simulink model "Copy_of_fast_powertrain"  (R2020b)
settings: Solver=FixedStepAuto  StartTime=0  StopTime=t(end)  RelTol=1e-3
PreLoadFcn:
  | C_sc = 1;
StartFcn:
  | C_sc = 1;
values from neighbouring files (symbols this model uses):
  fc_power_array = [900 900 900 900 900 900 900 900 900 900 900 900 ... (24566 elements, 71x346)]    [fc_power_climb_dp.mat]    (also in fc_power_cruise_dp.mat = [0 0 0 0 0 0 0 0 0 0 0 0 ... (32589 elements, 71x459)]; fc_power_descend_dp.mat = [285.411057245 285.411057245 285.411057245 285.411057245 285; fc_power_takeoff_dp.mat = [0 0 0 0 0 0 0 0 0 0 0 0 ... (23714 elements, 71x334)])
  Ts = old_data.Ts    [model_fc.m]
undefined symbols (not defined in the file or in its folder): DiscIntNeverNeededParam, Ion, Lithium, w
libraries: neural x50, powerlib x30, fuzblock x7, electricdrivelib x2, lib_converters x2, simulink x1
(part 1 of 5)
PostSaveFcn:
  | C_sc = 1;
settings Model: SimulationMode=accelerator  Creator=maloc  LastModifiedBy=maloc
settings DataIOCC: SaveOutput=off  SignalLogging=off  DSMLogging=off
settings OptimizationCC: StrengthReduction=on  PassReuseOutputArgsAs=Individual arguments  LocalBlockOutputs=off  ZeroExternalMemoryAtStartup=off  ZeroInternalMemoryAtStartup=off  OptimizeBlockOrder=speed  OptimizationPriority=Speed  MultiThreadedLoops=on  EfficientTunableParamExpr=on
settings DebuggingCC: RTPrefix=none  StringTruncationChecking=none  AlgebraicLoopMsg=none  ArtificialAlgebraicLoopMsg=none  MaxConsecutiveZCsMsg=none  InheritedTsInSrcMsg=none  MultiTaskDSMMsg=none  MultiTaskCondExecSysMsg=none  MultiTaskRateTransMsg=warning  TasksWithSamePriorityMsg=none  SigSpecEnsureSampleTimeMsg=none  IntegerOverflowMsg=none  Int32ToFloatConvMsg=none  ParameterDowncastMsg=none  ParameterOverflowMsg=none  ParameterPrecisionLossMsg=none  ParameterTunabilityLossMsg=none  FcnCallInpInsideContextMsg=warning  UnconnectedInputMsg=none  UnconnectedOutputMsg=none  UnconnectedLineMsg=none  FrameProcessingCompatibilityMsg=none  BusObjectLabelMismatch=none  RootOutportRequireBusObject=none  UnknownTsInhSupMsg=none  ModelReferenceDataLoggingMessage=none  ModelReferenceExtraNoncontSigs=none  OperatingPointInterfaceChecksumMismatchMsg=none  NonCurrentReleaseOperatingPointMsg=warning  SFUnexpectedBacktrackingDiag=warning  SFNoUnconditionalDefaultTransitionDiag=warning  IntegerSaturationMsg=none
settings SFSimCC: MATLABDynamicMemAlloc=off  SimTargetLang=C++
settings RTWCC: Description=Embedded Coder  SystemTargetFile=ert.tlc  GenCodeOnly=on  TemplateMakefile=ert_default_tmf  GenerateReport=on  BuildConfiguration=Debug  LaunchReport=on
settings CodeAppCC: ForceParamTrailComments=on  IgnoreCustomStorageClasses=off  OperatorAnnotations=on  SimulinkDataObjDesc=on  SFDataObjDesc=on  InsertBlockDesc=on  EnableCustomComments=on
settings ERTTargetCC: TargetLangStandard=C99 (ISO)  GenerateSampleERTMain=on  ERTCustomFileTemplate=example_file_process.tlc

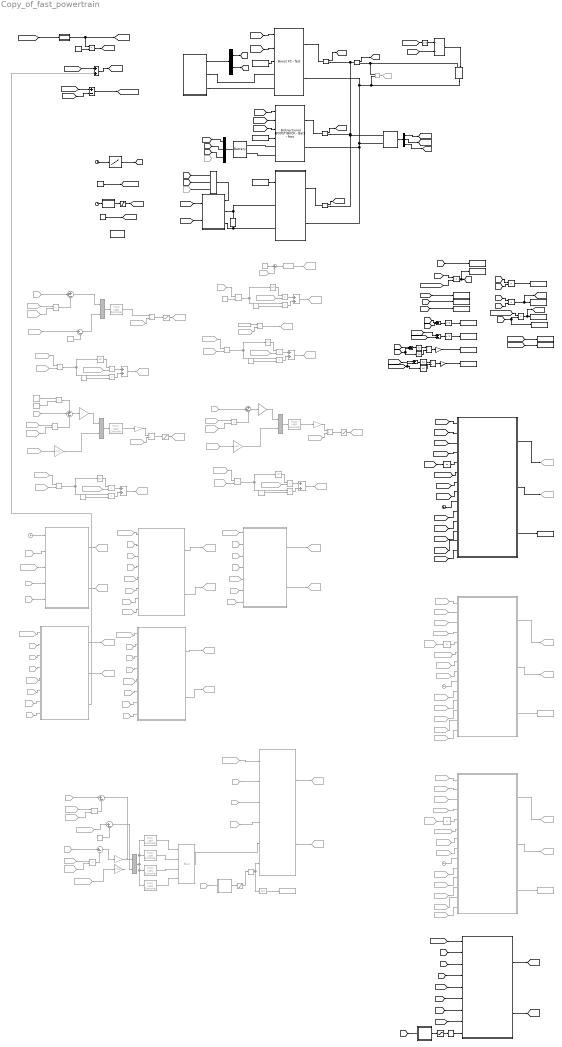
== system Copy_of_fast_powertrain ==
  note: GA
  note: DP-ANFIS
  note: Pload
  note: Data
  note: Powertrain
  note: Load
  note: Inputs
  note: BATT Control
  note: PV - FC Control
  note: PV Panel weather data
  note: ANFIS+NN
  1-D Lookup Table1 : Lookup_n-D  NumberOfTableDimensions=1  BreakpointsForDimension1=t  Table=w  InternalRulePriority=Speed  RndMeth=Simplest  InputSameDT=on
  Abs{,1..3} (4 alike) : Abs
  Battery : electricdrivelib/Extra Sources/Battery  BatType=Lithium-Ion  ShowTempParam=off  ThermalPreset=no  ShowAgeParam=off  NomV=48  NomQ=15  SOC=80  Batt_Tr=20  PresetModel=on  MaxQ=15  MinV=36  FullV=55.8714  Dis_rate=6.5217  R=0.032  Normal_OP=13.5652  expZone="[51.8585     0.736957]"  current=[2 5 10 40]  Units=Time  Tci=20  NomT=20  T2=-30  MaxQ2=4.8  FullV2=7.1  Normal_OP2=5.655  expZone2="[6.58           1]"  Rca=0.6  ti=2000  Dp=0  Neq0=0  Tsim=Ts  Ta1=25  Qeol=5.4*0.9  Reol=0.013333*1.2  Char_age=[2.3478, 3]  Dis_age=[2.3478, 10]  N1=1500  N2=10500  N3=1000  N4=1400  Ta2=45  N5=950
      link override Model/Constant15: Value=Batt_Tr
  Bidirectional BOOST/BUCK - Batt - fast : lib_converters/Bidirectional BOOST//BUCK - Batt - fast  n_buck=0.9  Tr_buck=1  damp_buck=0.707  n_boost=0.9  Tr_boost=1  damp_boost=0.707  max_curr=[30 -4]  Co=1e-4  CL=C_sc  Li=1e-3  Ts=Ts
  Boost - PV - fast : Subsystem  AncestorBlock=lib_converters/Boost - PV - fast  mask(Average value DC/DC boost converter for PV panel){n=0.9, Co=1e-4, CL=C_sc, Li=2e-3, damp=0.707, Tr=0.1, Ts=Ts}
      mask prompts: n "Efficiency [0,1]"; Co "Inside output capacitance (F)"; CL "Load Capacitance (F)"; Li "Input Inductor (H)"; damp "Damping ratio"; Tr "Response time (s) (Voltage Regulator)"; Ts "Sample time (s)"
      mask help:
      | This block implements an average-value DC/DC boost converter.
      | - VH* input is the control variable of the output voltage of the converter.
      | - IL*(max) input is the control variable of the input max current of the converter.
      | - I/O input control the converter to enable it to work or not (interruptor control command).
      | - Control input is the variable that manage the control strategy of the converter (MPPT, Cascade control, ...).
      mask init:
      | L=Li; 
      | C=Co+CL;
      | 
      | %Current regulator
      | zetai=damp;
      | thau_si=Tr/10;
      | zetawni=(-log(0.05*sqrt(1-zetai^2)))/thau_si;
      | Kpi=2*L*zetawni;
      | wni=zetawni/zetai;
      | Kii=L*wni^2;
      | 
      | %Voltage regulator
      | zetav=damp;
      | thau_sv=Tr; %response time
      | zetawnv=(-log(0.05*sqrt(1-zetav^2)))/thau_sv;
      | Kpv=2*C*zetawnv;
      | wnv=zetawnv/zetav;
      | Kiv=C*wnv^2;
      mask Help:
      | 1 - MPPT
      | 2 - Cascade control
  Boost FC - fast : lib_converters/Boost FC - fast  conv_type=Average model  n=0.9  Co=1e-4  CL=C_sc  Li=2e-3  damp=0.707  Tr=1  Ts=Ts
  Bus Selector : BusSelector  OutputSignals=SOC (%),Current (A),Voltage (V)
  Bus Selector1 : BusSelector  OutputSignals=Current I,SOC %,Voltage V
  Bus Selector2 : BusSelector  OutputSignals=Vout,Ifc
  Bus Selector3 : BusSelector  OutputSignals=V_PV,I_PV,Temperature (deg C)
  C2 : powerlib/Elements/Series RLC Branch  LConnTagsString=__new0  RConnTagsString=__new0  BranchType=C  Resistance=0.01  Inductance=1e-3  SetiL0=off  InitialCurrent=0  Capacitance=1e-3  Setx0=off  InitialVoltage=0  Measurements=None
  Clock : Clock  Commented=on
  Clock1 : Clock
  Clock2 : Clock  Commented=on
  Clock3 : Clock  Commented=on
  Clock4 : Clock
  Clock6 : Clock
  Constant : Constant  Commented=on  Value=20
  Constant1 : Constant
  Constant10 : Constant  Commented=on  Value=80
  Constant{4,11,13,17,19} (5 alike) : Constant  Commented=on  Value=100
  Constant14 : Constant  Commented=on  Value=20
  Constant15 : Constant  Commented=on  Value=180
  Constant16 : Constant  Commented=on  Value=0.9
  Constant2 : Constant
  Constant3 : Constant
  Constant5 : Constant  Commented=on  Value=580
  Constant6 : Constant  Value=72
  Constant7 : Constant  Commented=on  Value=80
  Constant8 : Constant  Value=0
  Constant9 : Constant  Value=25
  Current Measurement{,2..4} (4 alike) : powerlib/Measurements/Current Measurement  PhasorSimulation=off  OutputType=Complex  PSBequivalent=0
  DP : MATLAB Function  Commented=on  TreatAsAtomicUnit=on  mask{fc_power_array=fc_power_array}
  Discrete PI Controller1 : Subsystem  Commented=on  DialogController=POWERSYS.PowerSysDialog  mask(Discrete PI Controller){Kp=10, Ki=10, Par_Limits=[33 0], Init=0, Ts=Ts}
      mask prompts: Kp "Proportional gain (Kp):"; Ki "Integral gain (Ki):"; Par_Limits "Output limits: [ Upper   Lower ]"; Init "Output initial value:"; Ts "Sample time:"
      mask help: This block implements a discrete PI controller.
      mask init:
      | UpperLimit=Par_Limits(1);
      | LowerLimit=Par_Limits(2);
      | power_initmask();
      mask Help: This block is part of a subset of blocks in the Extras library that does not have documentation associated with it, other than the block mask description.
      mask Display: disp('PI');
  Discrete PI Controller2 : Subsystem  DialogController=POWERSYS.PowerSysDialog  mask(Discrete PI Controller){Kp=10, Ki=100, Par_Limits=[30 -4], Init=0, Ts=Ts}
      mask prompts: Kp "Proportional gain (Kp):"; Ki "Integral gain (Ki):"; Par_Limits "Output limits: [ Upper   Lower ]"; Init "Output initial value:"; Ts "Sample time:"
      mask help: This block implements a discrete PI controller.
      mask init:
      | UpperLimit=Par_Limits(1);
      | LowerLimit=Par_Limits(2);
      | power_initmask();
      mask Help: This block is part of a subset of blocks in the Extras library that does not have documentation associated with it, other than the block mask description.
      mask Display: disp('PI');
  Divide : Product  Inputs=*/
  Divide{1,4..6} (4 alike) : Product  Commented=on  Inputs=*/
  Divide2 : Product  Inputs=*/
  Divide3 : Product  Inputs=*/
  ECMS : MATLAB Function  Commented=on  TreatAsAtomicUnit=on
  EEDMS : MATLAB Function  Commented=on  TreatAsAtomicUnit=on
  EEMS : MATLAB Function  Commented=on  TreatAsAtomicUnit=on
  From100 : From  Commented=on  GotoTag=Vbus_real
  From{4,25,41,47,50,58,68,78,86,94,101,110,141} (13 alike) : From  Commented=on  GotoTag=V_dc_bus_wanted
  From{3,27,48,52,59,69,79,87,95,102,120,149} (12 alike) : From  Commented=on  GotoTag=V_fc
  From{26,38,49,53,60,70,76,84,92,103,118,123,147,150} (14 alike) : From  Commented=on  GotoTag=I_fc
  From{43,57,65,74,83,91,104,111,137,142} (10 alike) : From  Commented=on  GotoTag=V_dc_bus
  From105 : From  Commented=on  GotoTag=Vbus_real
  From106 : From  Commented=on  GotoTag=BATT_SOC
  From{39,54,61,71,81,89,96,98,107,113,139,152} (12 alike) : From  Commented=on  GotoTag=Pload
  From108 : From  Commented=on  GotoTag=Ipv_out
  From{42,56,64,73,82,90,109,136,140} (9 alike) : From  Commented=on  GotoTag=I_pv_out
  From{13,35,40,51,55,63,72,80,88,112,116,145} (12 alike) : From  Commented=on  GotoTag=SOC_batt
  From114 : From  Commented=on  GotoTag=I_fc_out
  From{34,77,85,93,115,144} (6 alike) : From  Commented=on  GotoTag=I_fc_conv
  From117 : From  Commented=on  GotoTag=Pfc_in
  From{66,75,119,148} (4 alike) : From  Commented=on  GotoTag=I_batt
  From138 : From  Commented=on  GotoTag=Pout
  From143 : From  Commented=on  GotoTag=I_fc_out
  From146 : From  Commented=on  GotoTag=Pfc_in
  From151 : From  Commented=on  GotoTag=Pout
  From67 : From  Commented=on  GotoTag=Pbatt_in
  From97 : From  Commented=on  GotoTag=BATT_SOC
  From99 : From  Commented=on  GotoTag=Ipv_out
  Fuzzy Logic Controller : fuzblock/Fuzzy Logic  Controller  Commented=on  FIS='DP_ANFIS_mid.fis'  OutputSampleNumber=10  DataType=double  FuzzifiedInputs=off  RuleFiringStrengths=off  RuleOutputs=off  AggregatedOutputs=off  SimulateUsing=Code generation  OutOfRangeInputValueMessage=warning  NoRuleFiredMessage=warning  EmptyOutputFuzzySetMessage=warning
  Fuzzy Logic Controller1 : fuzblock/Fuzzy Logic  Controller  Commented=on  FIS='fuzzy_for_final_1.fis'  OutputSampleNumber=10  DataType=double  FuzzifiedInputs=off  RuleFiringStrengths=off  RuleOutputs=off  AggregatedOutputs=off  SimulateUsing=Code generation  OutOfRangeInputValueMessage=warning  NoRuleFiredMessage=warning  EmptyOutputFuzzySetMessage=warning
  Fuzzy Logic Controller2 : fuzblock/Fuzzy Logic  Controller  Commented=on  FIS='fis_thesis_solo.fis'  OutputSampleNumber=10  DataType=double  FuzzifiedInputs=off  RuleFiringStrengths=off  RuleOutputs=off  AggregatedOutputs=off  SimulateUsing=Code generation  OutOfRangeInputValueMessage=warning  NoRuleFiredMessage=warning  EmptyOutputFuzzySetMessage=warning
  Goto{13,25,28,30,32,34,39..41,44,47,49,51,55} (14 alike) : Goto  Commented=on  GotoTag=V_fc_conv
  Goto{7,24,27,29,31,33,37,42..43,45..46,48,50,54} (14 alike) : Goto  Commented=on  GotoTag=I_fc_conv
  Goto36 : Goto  Commented=on  GotoTag=T_pv
  Goto38 : Goto  Commented=on  GotoTag=Age
  Goto53 : Goto  Commented=on  GotoTag=V_dc_bus
  GreaterThan{,2..5} (5 alike) : RelationalOperator  Commented=on  Operator=<  OutDataTypeStr=boolean  RndMeth=Simplest
  GreaterThan1 : RelationalOperator  Operator=<  OutDataTypeStr=boolean  RndMeth=Simplest
  LMC : MATLAB Function  TreatAsAtomicUnit=on
  LMC-deep : MATLAB Function  Commented=on  TreatAsAtomicUnit=on
  LMC-deep1 : MATLAB Function  Commented=on  TreatAsAtomicUnit=on
  Multiply : Gain  Gain=100
  Multiply1 : Gain  Gain=100
  Multiply2 : Gain  Commented=on  Gain=1/1550
  Multiply3 : Gain  Commented=on  Gain=1/100
  Multiply4 : Gain  Commented=on  Gain=1100
  Multiply5 : Gain  Commented=on  Gain=1/1550
  Multiply6 : Gain  Commented=on  Gain=1/100
  Multiply7 : Gain  Commented=on  Gain=1100
  Multiply8 : Gain  Commented=on  Gain=1/1500
  Multiply9 : Gain  Commented=on  Gain=1/100
  Mux{,1..3} (4 alike) : Mux  Commented=on  Inputs=2
  Mux4 : Mux  Commented=on
      settings: DisplayOption=signals
  NN-SMC : MATLAB Function  TreatAsAtomicUnit=on
  NOT{,1..4} (5 alike) : Logic  Commented=on  Operator=NOT  IconShape=distinctive  AllPortsSameDT=off  OutDataTypeStr=boolean
  PEMFC matfunc V1 : Subsystem  mask{P_H2=0.5, P_O2=1, T=313.15, W=14, tm=1.27e-4, Nfc=50, Rohm=0.061871, Ts=Ts, fc_tau=1}
      mask prompts: P_H2 "Hydrogen pressure (atm)"; P_O2 "Oxygen pressure (atm)"; T "Temperature (K)"; W "Water Content"; tm "Thickness of the membrane (m)"; Nfc "Number of cells"; Rohm "Fuel cell resistance"; Ts "Sample time (s)"; fc_tau "Dynamic response of the FC (s)"
      mask init:
      | tau = fc_tau / 5;
  PV - FC - control1 : MATLAB Function  Commented=on  TreatAsAtomicUnit=on
  PV MODULE2 : Subsystem  mask{Npar=1, Nser=1, Ncell=72, Pm=0, Voc=44.5, Isc=5.54, Vmpp=37.2, Impp=4.97, beta_Voc_pc=-0.34, alpha_Isc_pc=-0.017, beta_Voc=0, alpha_Isc=0, IL=5.55564, I0=2.39143e-10, df=0.96618, Rsh=113.762, Rs=0.32122, Ts=Ts}
      mask prompts: Npar "Parallel connected modules"; Nser "Series connected modules"; Ncell "Number of cells per module"; Pm "Maxium Power (W)"; Voc "Open circuit voltage Voc (V)"; Isc "Short-circuit current Isc (A)"; Vmpp "Voltage at MPP (V)"; Impp "Current at MPP (A)"; beta_Voc_pc "Temperature coefficient of Voc (%/deg.C"; alpha_Isc_pc "Temperature coefficient of Isc (%/deg.C)"; beta_Voc "Temperature coefficient of Voc (V/deg.C)"; alpha_Isc "Temperature coefficient of Isc (A/deg.C)"; IL "Light-generated current IL (A)"; I0 "Diode saturation current I0 (A)"; df "Diode ideality factor"; Rsh "Shunt resistance Rsh (ohms)"; Rs "Series resistance Rs (ohms)"; Ts "Sample time (s)"
      mask init:
      | if alpha_Isc ~= 0
      |     alpha = alpha_Isc;
      | else 
      |     alpha = alpha_Isc_pc * Isc/100;
      | end
      mask DialogControl Container5 Prompt: Module data
      mask DialogControl Container3 Prompt: Data from data sheet
      mask DialogControl Container6 Prompt: Data from NREL
  Product{,1,4,7} (4 alike) : Product
  Product{2..3,5..6,8..18,21} (16 alike) : Product  Commented=on
  Round : Rounding  Commented=on  Operator=round
  Round1 : Rounding  Operator=round
  SMC : MATLAB Function  Commented=on  TreatAsAtomicUnit=on
  Saturation : Saturate  UpperLimit=1000  LowerLimit=0
  Saturation1 : Saturate  Commented=on  UpperLimit=1100  LowerLimit=0
  Saturation2 : Saturate  Commented=on  UpperLimit=1100  LowerLimit=0
  Saturation3 : Saturate  Commented=on  UpperLimit=1100  LowerLimit=0
  Saturation4 : Saturate  Commented=on  UpperLimit=4  LowerLimit=1
  Saturation5 : Saturate  UpperLimit=4  LowerLimit=1
  Square : Math  Operator=square  SaturateOnIntegerOverflow=on
  Square1 : Math  Operator=square  SaturateOnIntegerOverflow=on
  Square2 : Math  Operator=square  SaturateOnIntegerOverflow=on
  Subsystem : Subsystem  Variant=on  VariantControlMode=label  VariantControl=Choice  LabelModeActiveChoice=Constant  mask{Choice=Constant, irradiance_const=800, irradiance1=[9.978198e-01,9.978198e-01,9.978198e-01], break1=[0,30,60], irradiance_step_init=1000, irradiance_step_end=500, break_step=5}
      mask prompts: Choice "Choose the model"; irradiance_const "Irradiance (W/m2)"; irradiance1 "Irradiance (W/m2)"; break1 "Time (s)"; irradiance_step_init "Irradiance init (W/m2)"; irradiance_step_end "Irradiance end (W/m2)"; break_step "Step Time (s)"
      mask init:
      | %Choose between control type
      | SimulinkModel  = [gcb,'/'];
      | 
      | switch Choice
      |     case 'Constant'
      |         set_param(gcb,'OverrideUsingVariant','Constant');
      |         
      |     case 'Step'
      |         set_param(gcb,'OverrideUsingVariant','Step');
      |         
      |     case 'Model-1'
      |         set_param(gcb,'OverrideUsingVariant','Model1');
      | end
      mask TypeOptions Choice: Constant | Step | Model-1
      mask DialogControl Container7 Prompt: Choose type irradiance model
      mask DialogControl Container5 Prompt: Constant
      mask DialogControl Container3 Prompt: Irradiance model 1
      mask DialogControl Container4 Prompt: Irradiance step
  Sum{,7,10,12..13} (5 alike) : Sum  Commented=on
  Sum{1..4,6} (5 alike) : Sum  Inputs=+-
  Sum{8,11,16..18} (5 alike) : Sum  Commented=on  Inputs=|+-
  Sum14 : Sum  Commented=on  Inputs=++-
  Sum15 : Sum  Commented=on  Inputs=++-
  Sum5 : Sum  Commented=on  Inputs=++-
  Sum9 : Sum
  Supercapacitor1 : electricdrivelib/Extra Sources/Supercapacitor  C=C_sc  Rdc=150e-3  Voltage=72  Ns=50  Np=1  Vinit=72  Temp=25  PresetModel=on  EstParam=off  Nc=1  r=1e-9  epsilon=6.0208e-10  Ich=10  Vstern="[0.161  2.7  7.8]"  Self_dis=on  Ioc=10  Vself="[48  47.8  47.06  44.65]"  demandeplot=off  I="[10  20 100  500]"  Units=sec  Vmax=0  If=0  deltaV=0.3  alpha=0.3  sec=0
      settings: SourceProductBaseCode=PS
  Time Delay Neural Network1 : Subsystem  Commented=on  mask{pi_input_1_delayed_1=0, pi_input_1_delayed_2=0, pi_input_1_delayed_3=0, pi_input_1_delayed_4=0, pi_input_1_delayed_5=0, pi_input_1_delayed_6=0, pi_input_1_delayed_7=0, pi_input_1_delayed_8=0, pi_input_1_delayed_9=0, pi_input_1_delayed_10=0, pi_input_1_delayed_11=0, pi_input_1_delayed_12=0, pi_input_1_delayed_13=0, pi_input_1_delayed_14=0, pi_input_1_delayed_15=0, pi_input_1_delayed_16=0, pi_input_1_delayed_17=0, pi_input_1_delayed_18=0, pi_input_1_delayed_19=0, pi_input_1_delayed_20=0}
      mask prompts: pi_input_1_delayed_1 "Preprocessed initial input 1 state at timestep 0."; pi_input_1_delayed_2 "Preprocessed initial input 1 state at timestep -1."; pi_input_1_delayed_3 "Preprocessed initial input 1 state at timestep -2."; pi_input_1_delayed_4 "Preprocessed initial input 1 state at timestep -3."; pi_input_1_delayed_5 "Preprocessed initial input 1 state at timestep -4."; pi_input_1_delayed_6 "Preprocessed initial input 1 state at timestep -5."; pi_input_1_delayed_7 "Preprocessed initial input 1 state at timestep -6."; pi_input_1_delayed_8 "Preprocessed initial input 1 state at timestep -7."; pi_input_1_delayed_9 "Preprocessed initial input 1 state at timestep -8."; pi_input_1_delayed_10 "Preprocessed initial input 1 state at timestep -9."; pi_input_1_delayed_11 "Preprocessed initial input 1 state at timestep -10."; pi_input_1_delayed_12 "Preprocessed initial input 1 state at timestep -11."; pi_input_1_delayed_13 "Preprocessed initial input 1 state at timestep -12."; pi_input_1_delayed_14 "Preprocessed initial input 1 state at timestep -13."; pi_input_1_delayed_15 "Preprocessed initial input 1 state at timestep -14."; pi_input_1_delayed_16 "Preprocessed initial input 1 state at timestep -15."; pi_input_1_delayed_17 "Preprocessed initial input 1 state at timestep -16."; pi_input_1_delayed_18 "Preprocessed initial input 1 state at timestep -17."; pi_input_1_delayed_19 "Preprocessed initial input 1 state at timestep -18."; pi_input_1_delayed_20 "Preprocessed initial input 1 state at timestep -19."
      mask help: Time Delay Neural Network
      mask Display: e = 0.06;c1 = [120 150 230]/255;c2 = ([120 150 230]+0)/383;c3 = ([120 150 230]+128)/383;patch([0 1 1 0],[0 0 1 1],c1);patch([0 1 1 1-e 1-e 0+e],[0 0 1 1-e 0+e 0+e],c2);patch([0 0 1 1-e 0+e 0+e],[0 1 1 1-e 1-e 0+e],c3);plot([0 1 1 0 0],[0 0 1 1 0]);fprintf('NNET');port_label('input',1,' x');port_label('output',1,'y ');
  Time Delay Neural Network2 : Subsystem  mask{pi_input_1_delayed_1=0, pi_input_1_delayed_2=0, pi_input_1_delayed_3=0, pi_input_1_delayed_4=0, pi_input_1_delayed_5=0, pi_input_1_delayed_6=0, pi_input_1_delayed_7=0, pi_input_1_delayed_8=0, pi_input_1_delayed_9=0, pi_input_1_delayed_10=0, pi_input_1_delayed_11=0, pi_input_1_delayed_12=0, pi_input_1_delayed_13=0, pi_input_1_delayed_14=0, pi_input_1_delayed_15=0, pi_input_1_delayed_16=0, pi_input_1_delayed_17=0, pi_input_1_delayed_18=0, pi_input_1_delayed_19=0, pi_input_1_delayed_20=0}
      mask prompts: pi_input_1_delayed_1 "Preprocessed initial input 1 state at timestep 0."; pi_input_1_delayed_2 "Preprocessed initial input 1 state at timestep -1."; pi_input_1_delayed_3 "Preprocessed initial input 1 state at timestep -2."; pi_input_1_delayed_4 "Preprocessed initial input 1 state at timestep -3."; pi_input_1_delayed_5 "Preprocessed initial input 1 state at timestep -4."; pi_input_1_delayed_6 "Preprocessed initial input 1 state at timestep -5."; pi_input_1_delayed_7 "Preprocessed initial input 1 state at timestep -6."; pi_input_1_delayed_8 "Preprocessed initial input 1 state at timestep -7."; pi_input_1_delayed_9 "Preprocessed initial input 1 state at timestep -8."; pi_input_1_delayed_10 "Preprocessed initial input 1 state at timestep -9."; pi_input_1_delayed_11 "Preprocessed initial input 1 state at timestep -10."; pi_input_1_delayed_12 "Preprocessed initial input 1 state at timestep -11."; pi_input_1_delayed_13 "Preprocessed initial input 1 state at timestep -12."; pi_input_1_delayed_14 "Preprocessed initial input 1 state at timestep -13."; pi_input_1_delayed_15 "Preprocessed initial input 1 state at timestep -14."; pi_input_1_delayed_16 "Preprocessed initial input 1 state at timestep -15."; pi_input_1_delayed_17 "Preprocessed initial input 1 state at timestep -16."; pi_input_1_delayed_18 "Preprocessed initial input 1 state at timestep -17."; pi_input_1_delayed_19 "Preprocessed initial input 1 state at timestep -18."; pi_input_1_delayed_20 "Preprocessed initial input 1 state at timestep -19."
      mask help: Time Delay Neural Network
      mask Display: e = 0.06;c1 = [120 150 230]/255;c2 = ([120 150 230]+0)/383;c3 = ([120 150 230]+128)/383;patch([0 1 1 0],[0 0 1 1],c1);patch([0 1 1 1-e 1-e 0+e],[0 0 1 1-e 0+e 0+e],c2);patch([0 0 1 1-e 0+e 0+e],[0 1 1 1-e 1-e 0+e],c3);plot([0 1 1 0 0],[0 0 1 1 0]);fprintf('NNET');port_label('input',1,' x');port_label('output',1,'y ');
  To Workspace : ToWorkspace  Commented=on  VariableName=pw_ph  SaveFormat=Timeseries  SampleTime=-1
  To Workspace1 : ToWorkspace  VariableName=RMSE_power  SaveFormat=Structure  SampleTime=-1
      settings: Save2DSignal=2-D array (concatenate along first dimension)
  To Workspace10 : ToWorkspace  VariableName=Pout_real  SaveFormat=Structure  SampleTime=-1
      settings: Save2DSignal=2-D array (concatenate along first dimension)
  To Workspace11 : ToWorkspace  VariableName=error_power  SaveFormat=Structure  SampleTime=-1
      settings: Save2DSignal=2-D array (concatenate along first dimension)
  To Workspace12 : ToWorkspace  VariableName=error_voltage  SaveFormat=Structure  SampleTime=-1
      settings: Save2DSignal=2-D array (concatenate along first dimension)
  To Workspace13 : ToWorkspace  VariableName=Pout_wanted  SaveFormat=Structure  SampleTime=-1
      settings: Save2DSignal=2-D array (concatenate along first dimension)
  To Workspace14 : ToWorkspace  VariableName=Ibatt  SaveFormat=Structure  SampleTime=-1
      settings: Save2DSignal=2-D array (concatenate along first dimension)
  To Workspace15 : ToWorkspace  VariableName=Vfc  SaveFormat=Structure  SampleTime=-1
      settings: Save2DSignal=2-D array (concatenate along first dimension)
  To Workspace16 : ToWorkspace  Commented=on  VariableName=gcf1  SaveFormat=Structure  SampleTime=-1
      settings: Save2DSignal=2-D array (concatenate along first dimension)
  To Workspace17 : ToWorkspace  VariableName=gcf  SaveFormat=Structure  SampleTime=-1
      settings: Save2DSignal=2-D array (concatenate along first dimension)
  To Workspace18 : ToWorkspace  Commented=on  VariableName=gcf2  SaveFormat=Structure  SampleTime=-1
      settings: Save2DSignal=2-D array (concatenate along first dimension)
  To Workspace2 : ToWorkspace  VariableName=RMSE_voltage  SaveFormat=Structure  SampleTime=-1
      settings: Save2DSignal=2-D array (concatenate along first dimension)
  To Workspace3 : ToWorkspace  VariableName=Ifc  SaveFormat=Structure  SampleTime=-1
      settings: Save2DSignal=2-D array (concatenate along first dimension)
  To Workspace4 : ToWorkspace  VariableName=SOC_batt  SaveFormat=Structure  SampleTime=-1
      settings: Save2DSignal=2-D array (concatenate along first dimension)
  To Workspace5 : ToWorkspace  VariableName=Vdc_wanted  SaveFormat=Structure  SampleTime=-1
      settings: Save2DSignal=2-D array (concatenate along first dimension)
  To Workspace6 : ToWorkspace  VariableName=Vdc_real  SaveFormat=Structure  SampleTime=-1
      settings: Save2DSignal=2-D array (concatenate along first dimension)
  To Workspace7 : ToWorkspace  VariableName=Ppv_in  SaveFormat=Structure  SampleTime=-1
      settings: Save2DSignal=2-D array (concatenate along first dimension)
  To Workspace8 : ToWorkspace  VariableName=Pbatt_in  SaveFormat=Structure  SampleTime=-1
      settings: Save2DSignal=2-D array (concatenate along first dimension)
  To Workspace9 : ToWorkspace  VariableName=Pfc_in  SaveFormat=Structure  SampleTime=-1
      settings: Save2DSignal=2-D array (concatenate along first dimension)
  Unit Delay1 : UnitDelay  Commented=on  SampleTime=-1  HasFrameUpgradeWarning=on
  Unit Delay2 : UnitDelay  Commented=on  SampleTime=-1  HasFrameUpgradeWarning=on
  Unit Delay3 : UnitDelay  SampleTime=-1  HasFrameUpgradeWarning=on
  Variable Resistor : powerlib/Elements/Variable Resistor  Rabsmin=1e-3
      settings: SourceProductBaseCode=PS
  Voltage Measurement : powerlib/Measurements/Voltage Measurement  Commented=on  PhasorSimulation=off  OutputType=Complex  PSBequivalent=0
  Zero-Order Hold : ZeroOrderHold  Commented=on  SampleTime=Ts
  climb : fuzblock/Fuzzy Logic  Controller  Commented=on  FIS='DP_ANFIS_climb.fis'  OutputSampleNumber=10  DataType=double  FuzzifiedInputs=off  RuleFiringStrengths=off  RuleOutputs=off  AggregatedOutputs=off  SimulateUsing=Code generation  OutOfRangeInputValueMessage=warning  NoRuleFiredMessage=warning  EmptyOutputFuzzySetMessage=warning
  cruise : fuzblock/Fuzzy Logic  Controller  Commented=on  FIS='DP_ANFIS_cruise.fis'  OutputSampleNumber=10  DataType=double  FuzzifiedInputs=off  RuleFiringStrengths=off  RuleOutputs=off  AggregatedOutputs=off  SimulateUsing=Code generation  OutOfRangeInputValueMessage=warning  NoRuleFiredMessage=warning  EmptyOutputFuzzySetMessage=warning
  descend : fuzblock/Fuzzy Logic  Controller  Commented=on  FIS='DP_ANFIS_descend.fis'  OutputSampleNumber=10  DataType=double  FuzzifiedInputs=off  RuleFiringStrengths=off  RuleOutputs=off  AggregatedOutputs=off  SimulateUsing=Code generation  OutOfRangeInputValueMessage=warning  NoRuleFiredMessage=warning  EmptyOutputFuzzySetMessage=warning
  powergui1 : powerlib/powergui  Priority=1  SimulationMode=Discrete  SampleTime=Ts  frequency=60  Iterations=50  frequencyindice=0  Pbase=100e6  ErrMax=1e-4  UnitsV=kV  UnitsW=MW  buscounter=0  FunctionMessages=off  echomessages=off  EnableUseOfTLC=off  CurrentSourceSwitches=off  DisableSnubberDevices=off  DisableRonSwitches=off  DisableVfSwitches=off  DisplayEquations=off  AutomaticDiscreteSolvers=off  SolverType=Tustin/Backward Euler (TBE)  Interpol=off  ExternalGateDelay=off  methode=off  Ts=100  x0status=blocks  SPID=on  SwTol=0  HookPort=off  NonlinearTolerance=1e-4  nMaxIteration=100  ContinueOnMaxIteration=off  RestoreLinks=warning  ResistiveCurrentMeasurement=off  Frange=[0:2:500]  Ylog=off  Xlog=on  ShowGrid=off  save=off  variable=ZData  structure=0  ZoomFFT=off  StartTime=0.0  cycles=1  DisplayStyle=1  fundamental=60  FreqAxis=off  MaxFrequency=1000  frequencyindicesteady=1  RmsSteady=1  display=off
  takeoff : fuzblock/Fuzzy Logic  Controller  Commented=on  FIS='DP_ANFIS_takeoff.fis'  OutputSampleNumber=10  DataType=double  FuzzifiedInputs=off  RuleFiringStrengths=off  RuleOutputs=off  AggregatedOutputs=off  SimulateUsing=Code generation  OutOfRangeInputValueMessage=warning  NoRuleFiredMessage=warning  EmptyOutputFuzzySetMessage=warning
  wires:
  Constant6/1 -> [V_dc_bus_wanted]  "Vbus_required"
  Battery/1 -> Bus Selector/1  "BATT"
  Current Measurement4/1 -> [I_fc_out]  "Ifc_output"
  Current Measurement3/1 -> [I_batt_out]  "Ibatt_output"
  Supercapacitor1/1 -> Bus Selector1/1
  Bus Selector/3 -> [V_batt]  "<Voltage (V)>"
  Bus Selector1/1 -> [I_sc]  "<Current I>"
  Current Measurement/1 -> [I_dc_bus]  "OUTPUT"
  Current Measurement2/1 -> [I_pv_out]  "Ibatt_output"
  Bus Selector/1 -> [SOC_batt]  "<SOC (%)>"
  [V_dc_bus_wanted] -> Square/1
  Square/1 -> Divide/1
  [Pload] -> Divide/2
  Divide/1 -> Variable Resistor/1
  Bus Selector1/2 -> [SOC_sc]  "<SOC %>"
  Clock6/1 -> 1-D Lookup Table1/1
  1-D Lookup Table1/1 -> [Pload]  "Pdemand"
  ? -> Goto38/1  "<Age (Equivalent Full cycles)>"
  From137/1 -> Product21/1
  [curr_batt_command_3] -> Discrete PI Controller2/1(Error)  "Batt current command 3"
  [V_dc_bus_wanted] -> Sum9/1
  From113/1 -> Sum5/2
  Product21/1 -> Sum5/3
  Mux/1 -> Fuzzy Logic Controller/1
  From136/1 -> Product21/2
  Sum5/1 -> Mux/1  "diff pload pdemand_fc"
  Bus Selector1/3 -> [V_dc_bus]  "<Voltage V>"
  Product/1 -> To Workspace10/1, [Pout]  "Pout_real"
  [I_dc_bus] -> Product/1
  [V_dc_bus] -> Product/2  "Vbus real"
  [SOC_batt] -> To Workspace4/1
  [Converter] -> Bidirectional BOOST/BUCK - Batt - fast/3
  [I_batt_conv] -> Bidirectional BOOST/BUCK - Batt - fast/2
  [V_batt_conv] -> Bidirectional BOOST/BUCK - Batt - fast/1
  Constant3/1 -> Bidirectional BOOST/BUCK - Batt - fast/4
  Constant2/1 -> Boost - PV - fast/1(I/O)
  Constant1/1 -> Boost FC - fast/3
  [I_fc_conv] -> Boost FC - fast/2
  From3/1 -> Divide1/2
  Discrete PI Controller1/1(Out) -> Goto7/1
  From35/1 -> GreaterThan/1
  GreaterThan/1 -> NOT/1, Product3/1
  Product2/1 -> Sum/1
  From4/1 -> Product2/2
  Sum/1 -> Goto13/1
  Product3/1 -> Sum/2
  Constant4/1 -> Product3/2
  NOT/1 -> Product2/1
  [V_dc_bus_wanted] -> Sum1/1
  [V_dc_bus] -> Sum1/2
  Sum1/1 -> [curr_batt_command_3]
  GreaterThan1/1 -> [Converter]
  Constant8/1 -> GreaterThan1/2
  Sum2/1 -> Square1/1
  [V_dc_bus] -> Sum3/1
  [Pout] -> Sum2/1
  [Pload] -> Sum2/2
  Sum3/1 -> Square2/1
  [V_dc_bus_wanted] -> Sum3/2
  Sum4/1 -> Abs1/1
  Abs1/1 -> Divide2/1
  Abs/1 -> Divide2/2
  Divide2/1 -> Multiply/1
  [Pload] -> Abs/1, Sum4/2
  [Pout] -> Sum4/1
  [V_dc_bus] -> Sum6/1
  [V_dc_bus_wanted] -> Abs2/1, Sum6/2
  Divide3/1 -> Multiply1/1
  Abs2/1 -> Divide3/2
  Abs3/1 -> Divide3/1
  Sum6/1 -> Abs3/1
  Square1/1 -> To Workspace1/1
  Square2/1 -> To Workspace2/1
  Multiply/1 -> To Workspace11/1
  Multiply1/1 -> To Workspace12/1
  Bus Selector/2 -> [I_batt]  "<Current (A)>"
  Discrete PI Controller2/1(Out) -> [I_batt_conv], GreaterThan1/1
  From112/1 -> Sum11/1
  [V_fc_conv] -> Boost FC - fast/1
  PEMFC matfunc V1/1(output) -> Bus Selector2/1
  Bus Selector2/1 -> [V_fc]  "<Vout>"
  Bus Selector2/2 -> [I_fc]  "<Ifc>"
  Bus Selector3/1 -> [V_pv]  "<V_PV>"
  PV MODULE2/1(data) -> Bus Selector3/1
  [CellTemp] -> PV MODULE2/1(TempCell_C)
  Bus Selector3/2 -> [I_pv]  "<I_PV>"
  [Irradiation] -> PV MODULE2/2(Irradiance)
  Bus Selector3/3 -> Goto36/1  "<Temperature (deg C)>"
  Clock4/1 -> Subsystem/1(In1)
  Subsystem/1(Out1) -> Saturation/1
  Constant9/1 -> [CellTemp]
  Saturation/1 -> [Irradiation]  "radiation"
  Constant7/1 -> GreaterThan/2
  [I_pv] -> Product1/1
  [V_pv] -> Product1/2
  Product1/1 -> To Workspace7/1  "P_pv_in"
  [I_batt] -> Product4/1
  [V_batt] -> Product4/2
  Product4/1 -> [Pbatt_in], To Workspace8/1  "P_batt_in"
  [I_fc] -> Product7/1  "FC"
  [V_fc] -> Product7/2, To Workspace15/1
  Product7/1 -> [Pfc_in], To Workspace9/1  "P_fc_in"
  From34/1 -> GreaterThan2/2
  From26/1 -> GreaterThan2/1
  From13/1 -> Sum8/2
  Constant10/1 -> Sum8/1
  Sum8/1 -> Discrete PI Controller1/1(Error)
  Constant5/1 -> Divide1/1
  Divide1/1 -> Goto24/1
  From25/1 -> SMC/1(Vdc_command)
  From27/1 -> SMC/2(Vfc)
  From38/1 -> SMC/3(Ifc_in)
  From39/1 -> SMC/4(Pload)
  From40/1 -> SMC/7(BATT_SOC)
  NOT1/1 -> Product5/1
  Constant11/1 -> Product6/2
  Product6/1 -> Sum7/2
  Sum7/1 -> Goto25/1
  From41/1 -> Product5/2
  Product5/1 -> Sum7/1
  GreaterThan2/1 -> Product6/1, NOT1/1
  SMC/2(Vfc_conv) -> Goto28/1
  SMC/1(Ifc) -> Goto27/1
  From42/1 -> SMC/5(I_pv_out)
  From43/1 -> SMC/6(Vdc_real)
  [V_dc_bus_wanted] -> To Workspace5/1
  [V_dc_bus] -> To Workspace6/1
  [Pload] -> To Workspace13/1
  DP/1(Ifc) -> Goto29/1
  DP/2(Vfc_conv) -> Goto30/1
  From51/1 -> DP/2(SOC_batt)
  From49/1 -> DP/4(Ifc_in)
  From47/1 -> DP/3(Vdc_command)
  Clock/1 -> DP/1(Time)
  From48/1 -> DP/5(Vfc)
  [I_fc] -> To Workspace3/1  "FC"
  [I_batt] -> To Workspace14/1
  From57/1 -> ECMS/6(Vdc_real)
  From56/1 -> ECMS/5(I_pv_out)
  ECMS/1(Ifc) -> Goto31/1
  ECMS/2(Vfc_conv) -> Goto32/1
  From55/1 -> ECMS/7(SOC)
  From54/1 -> ECMS/4(Pload)
  From53/1 -> ECMS/3(Ifc_in)
  From52/1 -> ECMS/2(Vfc)
  From50/1 -> ECMS/1(Vdc_command)
  From60/1 -> EEDMS/3(Ifc_in)
  From63/1 -> EEDMS/7(SOC)
  From61/1 -> EEDMS/4(Pload)
  From58/1 -> EEDMS/1(Vdc_command)
  EEDMS/1(Ifc) -> Goto33/1
  From64/1 -> EEDMS/5(I_pv_out)
  EEDMS/2(Vfc_conv) -> Goto34/1
  From59/1 -> EEDMS/2(Vfc)
  From65/1 -> EEDMS/6(Vdc_real)
  From66/1 -> EEDMS/8(Ibatt_in)
  From67/1 -> SMC/8(Pbatt_in)
  From75/1 -> EEMS/8(Ibatt_in)
  From74/1 -> EEMS/6(Vdc_real)
  From69/1 -> EEMS/2(Vfc)
  EEMS/2(Vfc_conv) -> Goto39/1
  From73/1 -> EEMS/5(I_pv_out)
  EEMS/1(Ifc) -> Goto37/1
  From68/1 -> EEMS/1(Vdc_command)
  From71/1 -> EEMS/4(Pload)
  From72/1 -> EEMS/7(SOC)
  From70/1 -> EEMS/3(Ifc_in)
  Sum9/1 -> [V_batt_conv]
  EEMS/3(DV) -> Sum9/2
  From76/1 -> GreaterThan3/1
  From78/1 -> Product9/2
  Product10/1 -> Sum10/2
  GreaterThan3/1 -> Product10/1, NOT2/1
  Sum10/1 -> Goto40/1
  NOT2/1 -> Product9/1
  Constant13/1 -> Product10/2
  From77/1 -> GreaterThan3/2
  Product9/1 -> Sum10/1
  Divide4/1 -> Saturation1/1
  Fuzzy Logic Controller/1 -> Divide4/1
  From79/1 -> Divide4/2
  Saturation1/1 -> Goto42/1
  Constant14/1 -> Sum11/2
  Sum11/1 -> Mux/2  "diff pload pdemand_fc"
  Divide5/1 -> Saturation2/1
  Multiply5/1 -> Mux1/1
  Saturation2/1 -> Goto43/1
  Product11/1 -> Sum12/2
  Constant16/1 -> Product13/2
  Product14/1 -> Sum12/1
  From85/1 -> GreaterThan4/2
  Sum12/1 -> Goto41/1
  Constant17/1 -> Product11/2
  Mux1/1 -> Fuzzy Logic Controller1/1
  From86/1 -> Product14/2
  From87/1 -> Divide5/2
  NOT3/1 -> Product14/1
  Multiply7/1 -> Divide5/1
  From81/1 -> Sum14/2
  From82/1 -> Product12/2
  Constant15/1 -> Product13/1
  Product13/1 -> Sum14/1
  From83/1 -> Product12/1
  Sum14/1 -> Multiply5/1  "diff pload pdemand_fc"
  Fuzzy Logic Controller1/1 -> Multiply7/1
  From80/1 -> Multiply6/1
  Product12/1 -> Sum14/3
  GreaterThan4/1 -> Product11/1, NOT3/1
  From84/1 -> GreaterThan4/1
  Multiply6/1 -> Mux1/2
  Sum15/1 -> Multiply2/1  "diff pload pdemand_fc"
  Multiply3/1 -> Mux2/2
  GreaterThan5/1 -> Product8/1, NOT4/1
  Mux2/1 -> Fuzzy Logic Controller2/1
  Multiply4/1 -> Divide6/1
  From92/1 -> GreaterThan5/1
  From90/1 -> Product15/2
  Fuzzy Logic Controller2/1 -> Multiply4/1
  From91/1 -> Product15/1
  Sum13/1 -> Goto44/1
  From89/1 -> Sum15/2
  Product15/1 -> Sum15/3
  NOT4/1 -> Product17/1
  From94/1 -> Product17/2
  Product8/1 -> Sum13/2
  Saturation3/1 -> Goto45/1
  Product17/1 -> Sum13/1
  From88/1 -> Multiply3/1
  Multiply2/1 -> Mux2/1
  Divide6/1 -> Saturation3/1
  From93/1 -> GreaterThan5/2
  From95/1 -> Divide6/2
  Constant19/1 -> Product8/2
  Saturation4/1 -> Round/1
  Zero-Order Hold/1 -> To Workspace/1
  Time Delay Neural Network1/1(y) -> Saturation4/1
  From99/1 -> Product16/2
  From100/1 -> Product16/1
  From98/1 -> Sum16/1
  Round/1 -> Zero-Order Hold/1, PV - FC - control1/6(NNres)  "classficiation power phase"
  cruise/1 -> Mux4/3  "cruise"
  Multiply9/1 -> ?
  descend/1 -> Mux4/4  "descend"
  Sum16/1 -> Multiply8/1  "diff pload pdemand_fc"
  Mux3/1 -> takeoff/1, climb/1, descend/1, cruise/1
  From96/1 -> Time Delay Neural Network1/1(x)
  PV - FC - control1/1(Ifc) -> Goto46/1
  From97/1 -> Multiply9/1
  Product16/1 -> Sum16/2
  PV - FC - control1/2(Vfc_conv) -> Goto47/1
  Mux4/1 -> PV - FC - control1/5(fuzzy_out)
  climb/1 -> Mux4/2  "climb"
  takeoff/1 -> Mux4/1  "takeoff"
  Multiply8/1 -> ?
  From101/1 -> PV - FC - control1/1(Vdc_command)
  From102/1 -> PV - FC - control1/2(Vfc)
  From103/1 -> PV - FC - control1/3(Ifc_in)
  From104/1 -> PV - FC - control1/4(Vdc_real)
  Product18/1 -> Sum17/2
  From106/1 -> Sum18/1
  Sum17/1 -> Mux3/1  "diff pload pdemand_fc"
  From107/1 -> Sum17/1
  From105/1 -> Product18/1
  From108/1 -> Product18/2
  Constant/1 -> Sum18/2
  Sum18/1 -> Mux3/2  "diff pload pdemand_fc"
  Clock1/1 -> LMC/9(t)
  [V_dc_bus_wanted] -> LMC/6(Vdc_ref)
  [I_pv_out] -> LMC/7(Ipv_out)
  [I_fc_out] -> LMC/4(Ifc_out)
  [I_fc_conv] -> Unit Delay3/1
  Unit Delay3/1 -> LMC/5(ILmax)
  [V_dc_bus] -> LMC/3(Vdc)
  LMC/1(Vfc_conv) -> Goto51/1  "Vfc_conv"
  LMC/2(Ifc_boost) -> Goto50/1  "Ifc_conv"
  [SOC_batt] -> LMC/8(SOC)
  [Pfc_in] -> LMC/10(Pfc_k)
  [I_fc] -> LMC/11(Ifc_in_k)
  [I_batt] -> LMC/12(Ibatt_in_k)
  LMC/3(f) -> To Workspace17/1  "Cost_func"
  [V_fc] -> LMC/1(Vfc)
  [I_fc] -> LMC/2(Ifc)
  [Pout] -> LMC/13(Pout_real)
  [Pload] -> LMC/14(Pwanted)
  Voltage Measurement/1 -> Goto53/1
  From139/1 -> LMC-deep/14(Pwanted)
  From138/1 -> LMC-deep/13(Pout_real)
  From123/1 -> LMC-deep/2(Ifc)
  From120/1 -> LMC-deep/1(Vfc)
  LMC-deep/3(f) -> To Workspace16/1  "Cost_func"
  From119/1 -> LMC-deep/12(Ibatt_in_k)
  From118/1 -> LMC-deep/11(Ifc_in_k)
  From117/1 -> LMC-deep/10(Pfc_k)
  From116/1 -> LMC-deep/8(SOC)
  LMC-deep/2(Ifc_boost) -> Goto48/1  "Ifc_conv"
  LMC-deep/1(Vfc_conv) -> Goto49/1  "Vfc_conv"
  From111/1 -> LMC-deep/3(Vdc)
  Unit Delay1/1 -> LMC-deep/5(ILmax)
  From115/1 -> Unit Delay1/1
  From114/1 -> LMC-deep/4(Ifc_out)
  From109/1 -> LMC-deep/7(Ipv_out)
  From110/1 -> LMC-deep/6(Vdc_ref)
  Clock2/1 -> LMC-deep/9(t)
  Clock3/1 -> LMC-deep1/9(t)
  From141/1 -> LMC-deep1/6(Vdc_ref)
  From140/1 -> LMC-deep1/7(Ipv_out)
  From143/1 -> LMC-deep1/4(Ifc_out)
  From144/1 -> Unit Delay2/1
  Unit Delay2/1 -> LMC-deep1/5(ILmax)
  From142/1 -> LMC-deep1/3(Vdc)
  LMC-deep1/1(Vfc_conv) -> Goto55/1  "Vfc_conv"
  LMC-deep1/2(Ifc_boost) -> Goto54/1  "Ifc_conv"
  From145/1 -> LMC-deep1/8(SOC)
  From146/1 -> LMC-deep1/10(Pfc_k)
  From147/1 -> LMC-deep1/11(Ifc_in_k)
  From148/1 -> LMC-deep1/12(Ibatt_in_k)
  LMC-deep1/3(f) -> To Workspace18/1  "Cost_func"
  From149/1 -> LMC-deep1/1(Vfc)
  From150/1 -> LMC-deep1/2(Ifc)
  From151/1 -> LMC-deep1/13(Pout_real)
  From152/1 -> LMC-deep1/14(Pwanted)
  [I_fc] -> NN-SMC/3(Ifc_in)
  [Pbatt_in] -> NN-SMC/8(Pbatt_in)
  [I_pv_out] -> NN-SMC/5(I_pv_out)
  [V_dc_bus] -> NN-SMC/6(Vdc_real)
  [SOC_batt] -> NN-SMC/7(BATT_SOC)
  NN-SMC/2(Vfc_conv) -> [V_fc_conv]
  [Pload] -> NN-SMC/4(Pload)
  NN-SMC/1(Ifc) -> [I_fc_conv]
  [V_dc_bus_wanted] -> NN-SMC/1(Vdc_command)
  [V_fc] -> NN-SMC/2(Vfc)
  Saturation5/1 -> Round1/1
  [Pload] -> Time Delay Neural Network2/1(x)
  Time Delay Neural Network2/1(y) -> Saturation5/1
  Round1/1 -> NN-SMC/9(nn_res)  "classficiation power phase"
  connections:
  Variable Resistor/LConn1 -- Voltage Measurement/LConn1 -- Current Measurement/RConn1
  Variable Resistor/RConn1 -- Voltage Measurement/LConn2 -- Boost - PV - fast/RConn2 -- Bidirectional BOOST/BUCK - Batt - fast/RConn2 -- Supercapacitor1/LConn2 -- Boost FC - fast/RConn2
  Current Measurement/LConn1 -- Current Measurement4/RConn1 -- Supercapacitor1/LConn1 -- Current Measurement2/RConn1 -- Current Measurement3/RConn1
  Bidirectional BOOST/BUCK - Batt - fast/LConn2 -- Battery/LConn2
  Bidirectional BOOST/BUCK - Batt - fast/LConn1 -- Battery/LConn1
  Bidirectional BOOST/BUCK - Batt - fast/RConn1 -- Current Measurement3/LConn1
  Boost FC - fast/RConn1 -- Current Measurement4/LConn1
  Boost - PV - fast/LConn2 -- PV MODULE2/RConn2 -- C2/RConn1
  Boost - PV - fast/RConn1 -- Current Measurement2/LConn1
  C2/LConn1 -- Boost - PV - fast/LConn1 -- PV MODULE2/RConn1
  PEMFC matfunc V1/RConn1 -- Boost FC - fast/LConn1
  PEMFC matfunc V1/RConn2 -- Boost FC - fast/LConn2

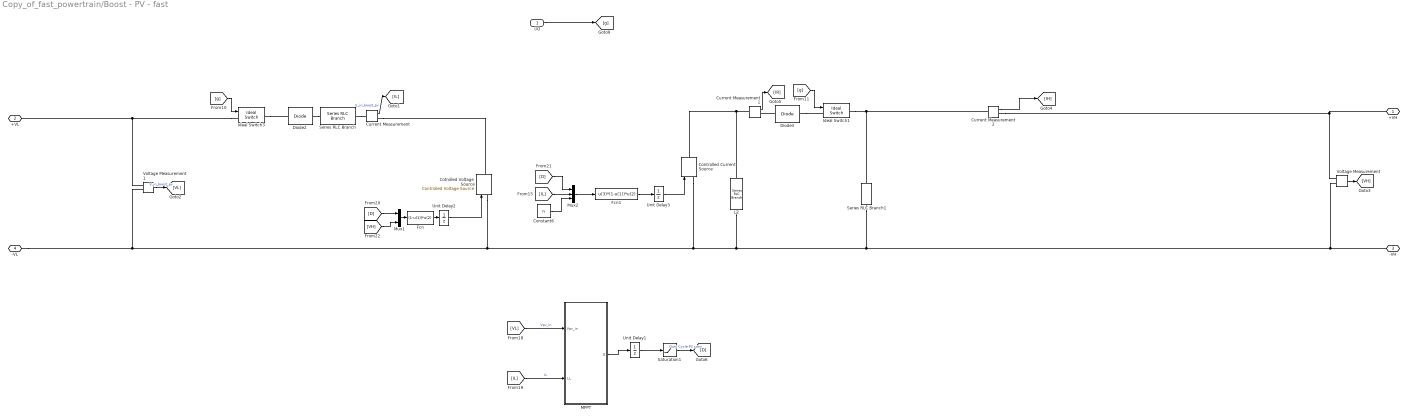
== system Copy_of_fast_powertrain/Boost - PV - fast ==
  I/O : Inport
  Constant6 : Constant  Value=n
  Controlled Current Source : powerlib/Electrical Sources/Controlled Current Source  Initialize=off  Source_Type=DC  Amplitude=0  Phase=0  Frequency=0  Measurements=None
  Cotrolled Voltage Source : powerlib/Electrical Sources/Controlled Voltage Source  Initialize=off  Source_Type=DC  Amplitude=0  Phase=0  Frequency=0  Measurements=None
  Current Measurement : powerlib/Measurements/Current Measurement  PhasorSimulation=off  OutputType=Complex  PSBequivalent=0
  Current Measurement1 : powerlib/Measurements/Current Measurement  PhasorSimulation=off  OutputType=Complex  PSBequivalent=0
  Current Measurement2 : powerlib/Measurements/Current Measurement  PhasorSimulation=off  OutputType=Complex  PSBequivalent=0
  Diode2 : powerlib/Power Electronics/Diode  Ron=0.001  Lon=0  Vf=0  IC=0  UseSnubber=off  Rs=1e6  Cs=250e-9  Measurements=off
  Diode3 : powerlib/Power Electronics/Diode  Ron=0.001  Lon=0  Vf=0  IC=0  UseSnubber=off  Rs=1e6  Cs=250e-9  Measurements=off
  Fcn : Fcn  Expr=(1-u(1))*u(2)
  Fcn1 : Fcn  Expr=u(3)*(1-u(1))*u(2)
  Ideal Switch1 : powerlib/Power Electronics/Ideal Switch  Ron=0.001  Lon=0  IC=0  Rs=1e5  Cs=inf  Measurements=off
  Ideal Switch3 : powerlib/Power Electronics/Ideal Switch  Ron=0.001  Lon=0  IC=0  Rs=1e5  Cs=inf  Measurements=off
  L2 : powerlib/Elements/Series RLC Branch  LConnTagsString=__new0  RConnTagsString=__new0  BranchType=C  Resistance=0.01  Inductance=100e-6  SetiL0=off  InitialCurrent=100  Capacitance=Co  Setx0=off  InitialVoltage=100  Measurements=None
  MPPT : MATLAB Function  TreatAsAtomicUnit=on
  Mux1 : Mux  Inputs=2
  Mux2 : Mux  Inputs=3
  Saturation1 : Saturate  UpperLimit=1  LowerLimit=0  SampleTime=Ts
  Series RLC Branch : powerlib/Elements/Series RLC Branch  LConnTagsString=__new0  RConnTagsString=__new0  BranchType=L  Resistance=1  Inductance=L  SetiL0=off  InitialCurrent=1  Capacitance=1e-6  Setx0=off  InitialVoltage=0  Measurements=None
  Series RLC Branch1 : powerlib/Elements/Series RLC Branch  LConnTagsString=__new0  RConnTagsString=__new0  BranchType=R  Resistance=5e3  Inductance=1e-3  SetiL0=off  InitialCurrent=0  Capacitance=15  Setx0=on  InitialVoltage=270  Measurements=None
  Unit Delay1 : UnitDelay  SampleTime=Ts*10  HasFrameUpgradeWarning=on
  Unit Delay2 : UnitDelay  SampleTime=Ts  HasFrameUpgradeWarning=on
  Unit Delay3 : UnitDelay  SampleTime=Ts  HasFrameUpgradeWarning=on
  Voltage Measurement : powerlib/Measurements/Voltage Measurement  PhasorSimulation=off  OutputType=Complex  PSBequivalent=0
  Voltage Measurement1 : powerlib/Measurements/Voltage Measurement  PhasorSimulation=off  OutputType=Complex  PSBequivalent=0
  +VH : PMIOPort  Side=Right
  +VL : PMIOPort  Port=2  Side=Left
  -VH : PMIOPort  Port=3  Side=Right
  -VL : PMIOPort  Port=4  Side=Left
  wires:
  Saturation1/1 -> [D]  "Duty Cycle PV conv"
  MPPT/1(D) -> Unit Delay1/1
  Unit Delay1/1 -> Saturation1/1
  I/O/1 -> [g]
  [IL] -> Mux2/2
  [VH] -> Mux1/2
  Unit Delay3/1 -> Controlled Current Source/1
  Voltage Measurement/1 -> [VH]
  [D] -> Mux2/1
  Fcn1/1 -> Unit Delay3/1
  Fcn/1 -> Unit Delay2/1
  [D] -> Mux1/1
  Mux2/1 -> Fcn1/1
  Constant6/1 -> Mux2/3
  Voltage Measurement1/1 -> [VL]  "V_in_boost_pv"
  Current Measurement1/1 -> [IR]
  Current Measurement/1 -> [IL]  "IL_in_boost_pv"
  Mux1/1 -> Fcn/1
  [g] -> Ideal Switch3/1
  [g] -> Ideal Switch1/1
  Unit Delay2/1 -> Cotrolled Voltage Source/1
  Current Measurement2/1 -> [IH]
  [VL] -> MPPT/1(Vpv_in)  "Vpv_in"
  [IL] -> MPPT/2(I_L)  "IL"
  connections:
  L2/LConn1 -- Controlled Current Source/RConn1 -- Current Measurement1/LConn1
  Ideal Switch3/LConn1 -- Voltage Measurement1/LConn1 -- +VL/RConn1
  Controlled Current Source/LConn1 -- L2/RConn1 -- -VH/RConn1 -- Voltage Measurement/LConn2 -- Series RLC Branch1/RConn1 -- Cotrolled Voltage Source/LConn1 -- Voltage Measurement1/LConn2 -- -VL/RConn1
  +VH/RConn1 -- Current Measurement2/RConn1 -- Voltage Measurement/LConn1
  Ideal Switch3/RConn1 -- Diode2/LConn1
  Diode2/RConn1 -- Series RLC Branch/LConn1
  Series RLC Branch/RConn1 -- Current Measurement/LConn1
  Current Measurement/RConn1 -- Cotrolled Voltage Source/RConn1
  Diode3/LConn1 -- Current Measurement1/RConn1
  Diode3/RConn1 -- Ideal Switch1/LConn1
  Ideal Switch1/RConn1 -- Current Measurement2/LConn1 -- Series RLC Branch1/LConn1

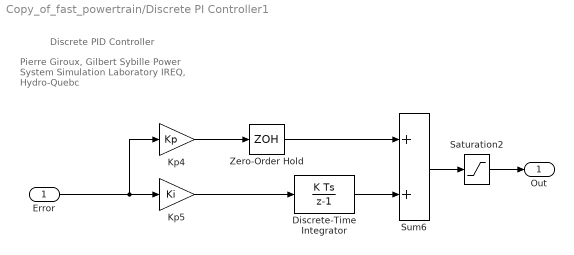
== system Copy_of_fast_powertrain/Discrete PI Controller1 ==
  note: Discrete PID Controller
  note: Pierre Giroux, Gilbert Sybille
      | Power System Simulation Laboratory
      | IREQ, Hydro-Quebc
  Error : Inport  SampleTime=Ts
  Discrete-Time Integrator : DiscreteIntegrator  InitialCondition=Init  SampleTime=Ts  LimitOutput=on  UpperSaturationLimit=UpperLimit  LowerSaturationLimit=LowerLimit  ICPrevOutput=DiscIntNeverNeededParam  ICPrevScaledInput=DiscIntNeverNeededParam
  Kp4 : Gain  Gain=Kp  SaturateOnIntegerOverflow=on  SampleTime=Ts  OutDataTypeStr=Inherit: Same as input  ParamDataTypeStr=Inherit: Same as input
  Kp5 : Gain  Gain=Ki  SaturateOnIntegerOverflow=on  SampleTime=Ts  OutDataTypeStr=Inherit: Same as input  ParamDataTypeStr=Inherit: Same as input
  Saturation2 : Saturate  UpperLimit=UpperLimit  LowerLimit=LowerLimit  SampleTime=Ts
  Sum6 : Sum  InputSameDT=on  SaturateOnIntegerOverflow=on  SampleTime=Ts  OutDataTypeStr=Inherit: Same as first input
  Zero-Order Hold : ZeroOrderHold  SampleTime=Ts
  Out : Outport  SampleTime=Ts  InitialOutput=0  VectorParamsAs1DForOutWhenUnconnected=off
  wires:
  Zero-Order Hold/1 -> Sum6/1
  Saturation2/1 -> Out/1
  Discrete-Time Integrator/1 -> Sum6/2
  Kp4/1 -> Zero-Order Hold/1
  Kp5/1 -> Discrete-Time Integrator/1
  Sum6/1 -> Saturation2/1
  Error/1 -> Kp5/1, Kp4/1

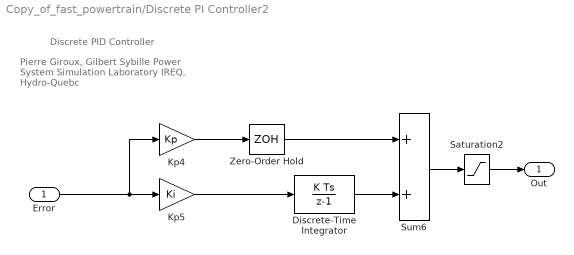
== system Copy_of_fast_powertrain/Discrete PI Controller2 ==
  note: Pierre Giroux, Gilbert Sybille
      | Power System Simulation Laboratory
      | IREQ, Hydro-Quebc
  note: Discrete PID Controller
  Error : Inport  SampleTime=Ts
  Discrete-Time Integrator : DiscreteIntegrator  InitialCondition=Init  SampleTime=Ts  LimitOutput=on  UpperSaturationLimit=UpperLimit  LowerSaturationLimit=LowerLimit  ICPrevOutput=DiscIntNeverNeededParam  ICPrevScaledInput=DiscIntNeverNeededParam
  Kp4 : Gain  Gain=Kp  SaturateOnIntegerOverflow=on  SampleTime=Ts  OutDataTypeStr=Inherit: Same as input  ParamDataTypeStr=Inherit: Same as input
  Kp5 : Gain  Gain=Ki  SaturateOnIntegerOverflow=on  SampleTime=Ts  OutDataTypeStr=Inherit: Same as input  ParamDataTypeStr=Inherit: Same as input
  Saturation2 : Saturate  UpperLimit=UpperLimit  LowerLimit=LowerLimit  SampleTime=Ts
  Sum6 : Sum  InputSameDT=on  SaturateOnIntegerOverflow=on  SampleTime=Ts  OutDataTypeStr=Inherit: Same as first input
  Zero-Order Hold : ZeroOrderHold  SampleTime=Ts
  Out : Outport  SampleTime=Ts  InitialOutput=0  VectorParamsAs1DForOutWhenUnconnected=off
  wires:
  Error/1 -> Kp4/1, Kp5/1
  Sum6/1 -> Saturation2/1
  Kp5/1 -> Discrete-Time Integrator/1
  Kp4/1 -> Zero-Order Hold/1
  Discrete-Time Integrator/1 -> Sum6/2
  Saturation2/1 -> Out/1
  Zero-Order Hold/1 -> Sum6/1
